simulink model "cmdGimbal"  (R2019b)
settings: Solver=FixedStepAuto  StartTime=0.0  StopTime=inf  FixedStep=0.001  RelTol=1e-3
libraries: lib_GRM_HIL x2, simulink x1, dspstat3 x1
settings Model: SimulationMode=external  Creator=m.hiepp  LastModifiedBy=guy-m
settings DataIOCC: SignalLogging=off  ReturnWorkspaceOutputs=off
settings DebuggingCC: ArithmeticOperatorsInVariantConditions=warning
settings SFSimCC: CustomCodeUndefinedFunction=UseInterfaceOnly
settings RTWCC: Description=Simulink Desktop Real-Time  SystemTargetFile=sldrt.tlc  TemplateMakefile=sldrt.tmf  RTWCompilerOptimization=on
settings CodeAppCC: MaxIdLength=95
settings SimulinkDesktopRealTimeCC: TargetPreCompLibLocation=C:\Program Files\MATLAB\R2019b\toolbox\sldrt\lib\win64  PreserveStateflowLocalDataDimensions=off

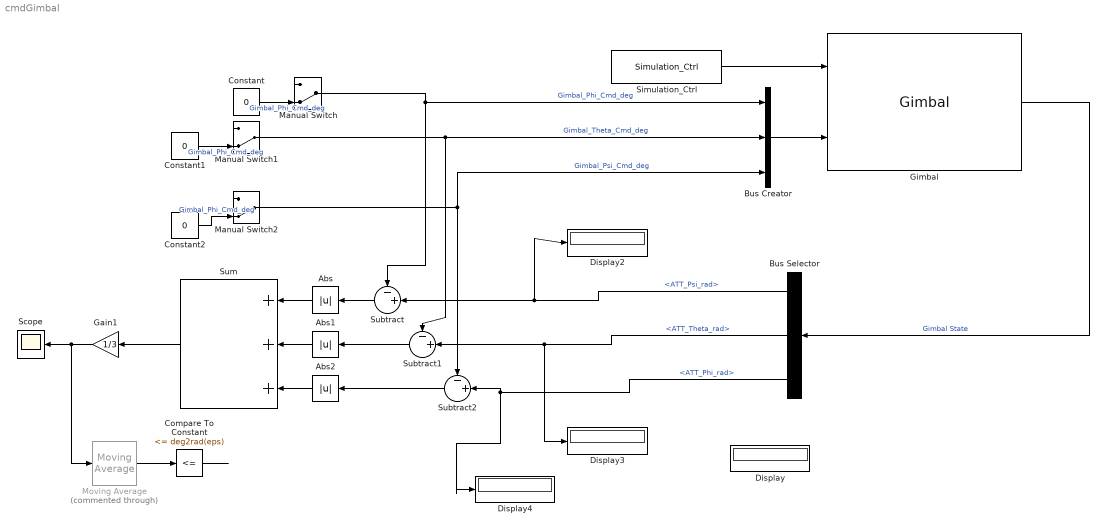
== system cmdGimbal ==
  Abs : Abs
  Abs1 : Abs
  Abs2 : Abs
  Bus Creator : BusCreator  Inputs=3  OutDataTypeStr=Bus: Gimbal_Cmd_Bus
  Bus Selector : BusSelector  OutputSignals=Gimbal_Attitude_Bus.ATT_Euler_Bus.ATT_Psi_rad,Gimbal_Attitude_Bus.ATT_Euler_Bus.ATT_Theta_rad,Gimbal_Attitude_Bus.ATT_Euler_Bus.ATT_Phi_rad
  Compare To Constant : simulink/Logic and Bit Operations/Compare To Constant  relop=<=  const=deg2rad(eps)  OutDataTypeStr=boolean
  Constant : Constant  Value=0
  Constant1 : Constant  Value=0
  Constant2 : Constant  Value=0
  Display{,2..4} (4 alike) : Display
      settings: Decimation=3
  Gain1 : Gain  Gain=1/3
  Gimbal : lib_GRM_HIL/Gimbal  SystemSampleTime=-1  Latency=0  AutoFrameSizeCalculation=off
  Manual Switch : ManualSwitch  CurrentSetting=0
  Manual Switch1 : ManualSwitch  CurrentSetting=0
  Manual Switch2 : ManualSwitch  CurrentSetting=0
  Moving Average : dspstat3/Moving Average  Commented=through  Method=Sliding window  ForgettingFactorPort=off  SpecifyWindowLength=on  WindowLength=100  ForgettingFactor=0.9  SimulateUsing=Code generation
  Scope : Scope
  Simulation_Ctrl : lib_GRM_HIL/Simulation_Ctrl  SystemSampleTime=-1  Latency=0  AutoFrameSizeCalculation=off
  Subtract : Sum  Inputs=-+|
  Subtract1 : Sum  Inputs=-+|
  Subtract2 : Sum  Inputs=-+|
  Sum : Sum  Inputs=+++
  wires:
  Simulation_Ctrl/1 -> Gimbal/1
  Manual Switch1/1 -> Bus Creator/2, Subtract1/1  "Gimbal_Theta_Cmd_deg"
  Bus Creator/1 -> Gimbal/2
  Manual Switch/1 -> Bus Creator/1, Subtract/1  "Gimbal_Phi_Cmd_deg"
  Manual Switch2/1 -> Bus Creator/3, Subtract2/1  "Gimbal_Psi_Cmd_deg"
  Gimbal/1 -> Bus Selector/1  "Gimbal State"
  Bus Selector/1 -> Display2/1, Subtract/2  "<ATT_Psi_rad>"
  Bus Selector/2 -> Display3/1, Subtract1/2  "<ATT_Theta_rad>"
  Bus Selector/3 -> Display4/1, Subtract2/2  "<ATT_Phi_rad>"
  Subtract/1 -> Abs/1
  Subtract1/1 -> Abs1/1
  Subtract2/1 -> Abs2/1
  Abs/1 -> Sum/1
  Abs1/1 -> Sum/2
  Abs2/1 -> Sum/3
  Sum/1 -> Gain1/1
  Gain1/1 -> Moving Average/1, Scope/1
  Compare To Constant/1 -> ?
  Moving Average/1 -> Compare To Constant/1
  Constant/1 -> Manual Switch/2  "Gimbal_Phi_Cmd_deg"
  ? -> Manual Switch/1
  ? -> Manual Switch1/1
  ? -> Manual Switch2/1
  Constant2/1 -> Manual Switch2/2  "Gimbal_Phi_Cmd_deg"
  Constant1/1 -> Manual Switch1/2  "Gimbal_Phi_Cmd_deg"
